simulink model "BEV_Model_DTCS_Project_Oral"  (R2022b)
settings: Solver=VariableStepAuto  StartTime=0.0  StopTime=1800  RelTol=1e-3
values from neighbouring files (symbols this model uses):
  d = struct('T1', 400, 'W1', 300, 'T2', 200, 'W2', 500, 'T3', 100, 'W3', 1000)    [Variables.m]
  dM = 6.5    [Variables.m]
  dr = 206    [Variables.m]
  F_L = cw*A*(Rho/2)    (= 0.3999)    [Variables.m]
  F_R = fr*vmass*g    (= 255.3543)    [Variables.m]
  I_veh_red = vmass * Rdyn^2 / itot^2    (= 1.18512110727)    [Variables.m]
  Imot = 0.9    [Variables.m]
  itot = 10.2    [Variables.m]
  Itrans = 1.2    [Variables.m]
  kM = 13000    [Variables.m]
  kr = 201.5    [Variables.m]
  lamba = 1+(mr/vmass)    (= 2.77197080292)    [Variables.m]
  Rdyn = 0.3    [Variables.m]
  vmass = 1370    [Variables.m]
libraries: slpidlib x1, simulink x1
settings Model: Creator=cogo  LastModifiedBy=cogo

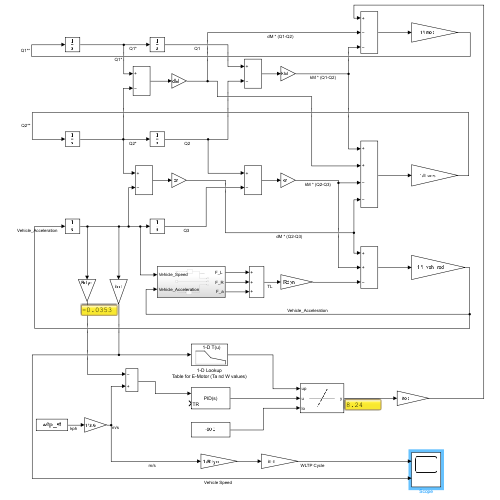
[thumbnail: Simulink's stored preview of the top-level diagram]
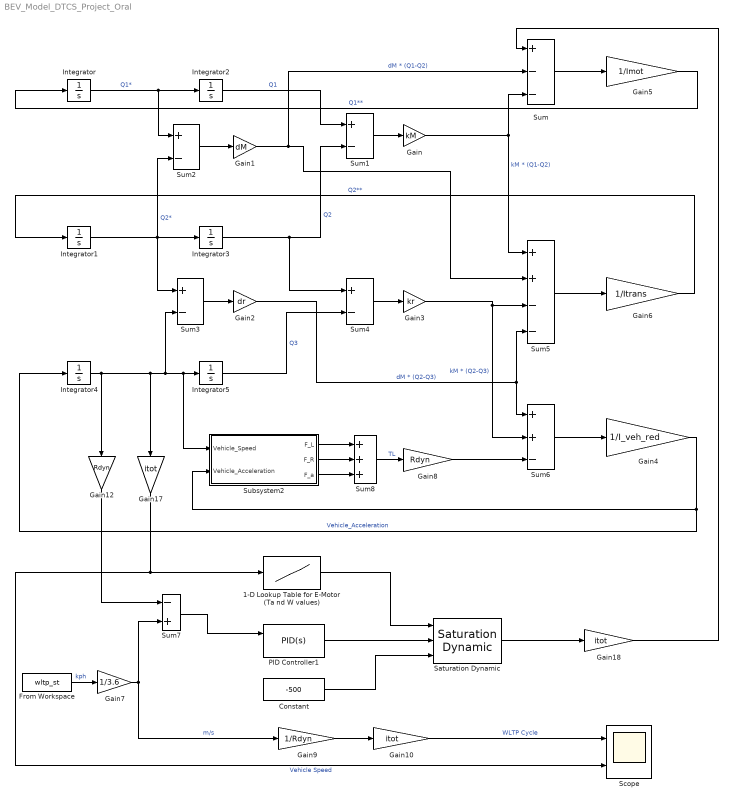
== system BEV_Model_DTCS_Project_Oral ==
  1-D Lookup Table for E-Motor (Ta nd W values) : Lookup_n-D  NumberOfTableDimensions=1  BreakpointsForDimension1=[0 d.W1 d.W2 d.W3 1000.1 1001]  Table=[d.T1 d.T1 d.T2 d.T3 0 0]  InternalRulePriority=Speed  RndMeth=Simplest
  Constant : Constant  Value=-500
  From Workspace : FromWorkspace  VariableName=wltp_st
  Gain : Gain  Gain=kM
  Gain1 : Gain  Gain=dM
  Gain10 : Gain  Gain=itot
  Gain12 : Gain  Gain=Rdyn
  Gain17 : Gain  Gain=itot
  Gain18 : Gain  Gain=itot
  Gain2 : Gain  Gain=dr
  Gain3 : Gain  Gain=kr
  Gain4 : Gain  Gain=1/I_veh_red
  Gain5 : Gain  Gain=1/Imot
  Gain6 : Gain  Gain=1/Itrans
  Gain7 : Gain  Gain=1/3.6
  Gain8 : Gain  Gain=Rdyn
  Gain9 : Gain  Gain=1/Rdyn
  Integrator{,1..5} (6 alike) : Integrator
  PID Controller1 : slpidlib/PID Controller  Controller=PID  Form=Parallel  TimeDomain=Continuous-time  UseExternalTs=off  SampleTime=-1  IntegratorMethod=Forward Euler  FilterMethod=Forward Euler  ControllerParametersSource=internal  P=2042.81894378046  I=7231.18124173872  UseKiTs=off  D=-10.266734007498  N=198.974566039069  UseFilter=on  TunerSelectOption=Transfer Function Based (PID Tuner App)  InitialConditionSource=internal  InitialConditionForIntegrator=0  InitialConditionForFilter=0  DifferentiatorICPrevScaledInput=0  ExternalReset=none  TrackingMode=on  Kt=1  LimitOutput=off  SatLimitsSource=internal  UpperSaturationLimit=inf  LowerSaturationLimit=-inf  LinearizeAsGain=on  AntiWindupMode=none  Kb=1  LimitIntegrator=off  UpperIntegratorSaturationLimit=inf  LowerIntegratorSaturationLimit=-inf  POutMin=[]  POutMax=[]  IOutMin=[]  IOutMax=[]  DOutMin=[]  DOutMax=[]  NOutMin=[]  NOutMax=[]  SumOutMin=[]  SumOutMax=[]  SaturationOutMin=[]  SaturationOutMax=[]  PParamMin=[]  PParamMax=[]  IParamMin=[]  IParamMax=[]  DParamMin=[]  DParamMax=[]  NParamMin=[]  NParamMax=[]  KbParamMin=[]  KbParamMax=[]  KtParamMin=[]  KtParamMax=[]  KbOutMin=[]  KbOutMax=[]  KtOutMin=[]  KtOutMax=[]  IntegratorOutMin=[]  IntegratorOutMax=[]  FilterOutMin=[]  FilterOutMax=[]  SumI1OutMin=[]  SumI1OutMax=[]  SumI2OutMin=[]  SumI2OutMax=[]  SumI3OutMin=[]  SumI3OutMax=[]  SumI4OutMin=[]  SumI4OutMax=[]  SumDOutMin=[]  SumDOutMax=[]  DifferentiatorOutMin=[]  DifferentiatorOutMax=[]  FilterDiffOutCoefMin=[]  FilterDiffOutCoefMax=[]  ReciprocalOutMin=[]  ReciprocalOutMax=[]  SumDenOutMin=[]  SumDenOutMax=[]  SumNumOutMin=[]  SumNumOutMax=[]  DivideOutMin=[]  DivideOutMax=[]  UdiffTsProdOutMin=[]  UdiffTsProdOutMax=[]  NTsProdOutMin=[]  NTsProdOutMax=[]  UintegralTsProdOutMin=[]  UintegralTsProdOutMax=[]  UngainTsProdOutMin=[]  UngainTsProdOutMax=[]  ClampingZeroOutDataTypeStr=Inherit: Inherit via back propagation  ClampingZeroOutMin=[]  ClampingZeroOutMax=[]  FilterDenConstantOutDataTypeStr=Inherit: Inherit via back propagation  FilterDenConstantOutMin=[]  FilterDenConstantOutMax=[]  PCopyOutDataTypeStr=Inherit: Inherit via back propagation  PCopyOutMin=[]  PCopyOutMax=[]  NCopyOutDataTypeStr=Inherit: Inherit via back propagation  NCopyOutMin=[]  NCopyOutMax=[]  IntegratorContinuousStateAttributes=''  IntegratorStateMustResolveToSignalObject=off  IntegratorRTWStateStorageClass=Auto  FilterContinuousStateAttributes=''  FilterStateMustResolveToSignalObject=off  FilterRTWStateStorageClass=Auto  ParallelPVariant=InternalParameters  IdealPVariant=Disabled  IVariant=InternalParameters  DVariant=InternalParameters  IntegratorVariant=Continuous  SatVariant=Disabled  AWVariant=Passthrough  PCopyVariant=Disabled  TRVariant=Enabled  FdbkBlocksVariant=Forward  IdealPFdbkVariant=Disabled  SatFdbkVariant=Disabled  DerivativeFilterVariant=ContFilter  NVariant=InternalParameters  NCopyVariant=Disabled  FilterICVariant=InternalICsFilter  IntegratorICVariant=InternalICs  ExternalResetVariant=Disabled  TRSumVariant=TrackingMode  SumFdbkVariant=Disabled  SumVariant=Sum_PID  TsampFilterVariant=InternalTs  TsampNgainVariant=Passthrough  TsampIntegralVariant=Passthrough  ExternalSaturationOutDataTypeStr=Inherit: Same as second input
  Saturation Dynamic : simulink/Discontinuities/Saturation Dynamic  OutMin=[]  OutMax=[]  OutDataTypeStr=Inherit: Same as second input  OutDataType=fixdt(1, 16)  OutScaling=2^-10  DoSatur=off
  Scope : Scope  NumInputPorts=2
  Subsystem2 : Subsystem
  Sum : Sum  Inputs=+--
  Sum{1..4} (4 alike) : Sum  Inputs=+-
  Sum5 : Sum  Inputs=++--
  Sum6 : Sum  Inputs=++-
  Sum7 : Sum  Inputs=-+
  Sum8 : Sum  Inputs=+++
  wires:
  Integrator/1 -> Integrator2/1, Sum2/1  "Q1*"
  Gain5/1 -> Integrator/1  "Q1**"
  Gain6/1 -> Integrator1/1  "Q2**"
  Integrator1/1 -> Sum3/1, Sum2/2, Integrator3/1  "Q2*"
  Gain4/1 -> Integrator4/1, Subsystem2/2(Vehicle_Acceleration)  "Vehicle_Acceleration"
  Integrator2/1 -> Sum1/1  "Q1"
  Integrator3/1 -> Sum4/1, Sum1/2  "Q2"
  Sum1/1 -> Gain/1
  Sum2/1 -> Gain1/1
  Gain/1 -> Sum/3, Sum5/1  "kM * (Q1-Q2)"
  Gain1/1 -> Sum5/2, Sum/2  "dM * (Q1-Q2)"
  Sum3/1 -> Gain2/1
  Integrator5/1 -> Sum4/2  "Q3"
  Gain2/1 -> Sum6/1, Sum5/4  "dM * (Q2-Q3)"
  Sum4/1 -> Gain3/1
  Gain3/1 -> Sum5/3, Sum6/2  "kM * (Q2-Q3)"
  Sum6/1 -> Gain4/1
  Sum/1 -> Gain5/1
  Sum5/1 -> Gain6/1
  From Workspace/1 -> Gain7/1  "kph"
  PID Controller1/1 -> Saturation Dynamic/2
  Gain7/1 -> Gain9/1, Sum7/2  "m/s"
  Sum7/1 -> PID Controller1/1
  Constant/1 -> Saturation Dynamic/3
  Sum8/1 -> Gain8/1  "TL"
  Integrator4/1 -> Subsystem2/1(Vehicle_Speed), Integrator5/1, Sum3/2, Gain17/1, Gain12/1
  Saturation Dynamic/1 -> Gain18/1
  Gain9/1 -> Gain10/1
  Gain8/1 -> Sum6/3
  Gain12/1 -> Sum7/1
  1-D Lookup Table for E-Motor (Ta nd W values)/1 -> Saturation Dynamic/1
  Gain17/1 -> Scope/2, 1-D Lookup Table for E-Motor (Ta nd W values)/1  "Vehicle Speed"
  Gain18/1 -> Sum/1
  Subsystem2/1("F_L ") -> Sum8/1
  Subsystem2/2(F_R) -> Sum8/2
  Subsystem2/3(F_a) -> Sum8/3
  Gain10/1 -> Scope/1  "WLTP Cycle"

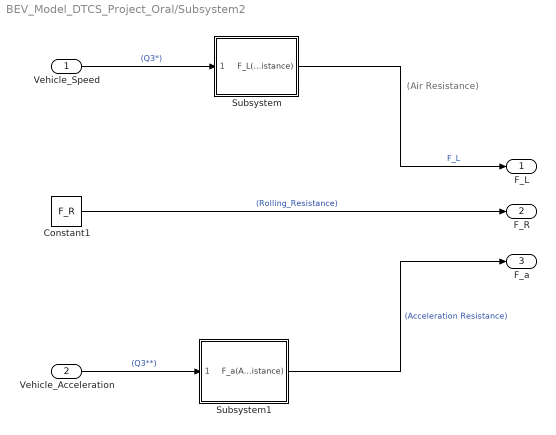
== system BEV_Model_DTCS_Project_Oral/Subsystem2 ==
  note: (Air Resistance)
  Vehicle_Speed : Inport
  Vehicle_Acceleration : Inport  Port=2
  Constant1 : Constant  Value=F_R
  Subsystem : Subsystem
  Subsystem1 : Subsystem
  "F_L " : Outport
  F_R : Outport  Port=2
  F_a : Outport  Port=3
  wires:
  Constant1/1 -> F_R/1  "(Rolling_Resistance)"
  Vehicle_Acceleration/1 -> Subsystem1/1(" ")  "(Q3**)"
  Subsystem1/1(F_a(Acc Resistance)) -> F_a/1  "(Acceleration Resistance)"
  Vehicle_Speed/1 -> Subsystem/1(" ")  "(Q3*)"
  Subsystem/1(F_L(Air Resistance)) -> "F_L "/1  "F_L"

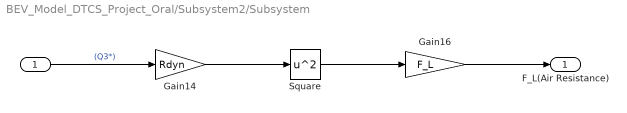
== system BEV_Model_DTCS_Project_Oral/Subsystem2/Subsystem ==
  " " : Inport
  Gain14 : Gain  Gain=Rdyn
  Gain16 : Gain  Gain=F_L
  Square : Math  Operator=square
  F_L(Air Resistance) : Outport
  wires:
  " "/1 -> Gain14/1  "(Q3*)"
  Square/1 -> Gain16/1
  Gain14/1 -> Square/1
  Gain16/1 -> F_L(Air Resistance)/1

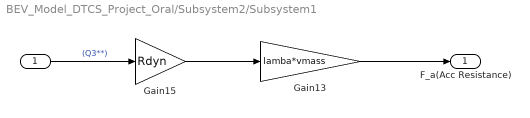
== system BEV_Model_DTCS_Project_Oral/Subsystem2/Subsystem1 ==
  " " : Inport
  Gain13 : Gain  Gain=lamba*vmass
  Gain15 : Gain  Gain=Rdyn
  F_a(Acc Resistance) : Outport
  wires:
  Gain13/1 -> F_a(Acc Resistance)/1
  Gain15/1 -> Gain13/1
  " "/1 -> Gain15/1  "(Q3**)"
